simulink model "mc2_current_speed_fuzzy"  (R2023b)
settings: Solver=ode45  StartTime=0.0  StopTime=12  MaxStep=1e-5  RelTol=1e-3
libraries: spsDCVoltageSourceLib x2, spsUniversalBridgeLib x2, spsVoltageMeasurementLib x2, simulink x2, fuzblock x1, spspowerguiLib x1, sps_lib x1
settings Model: Creator=86189  LastModifiedBy=86189
settings SolverCC: ZeroCrossAlgorithm=Adaptive
settings DebuggingCC: IgnoredZcDiagnostic=none

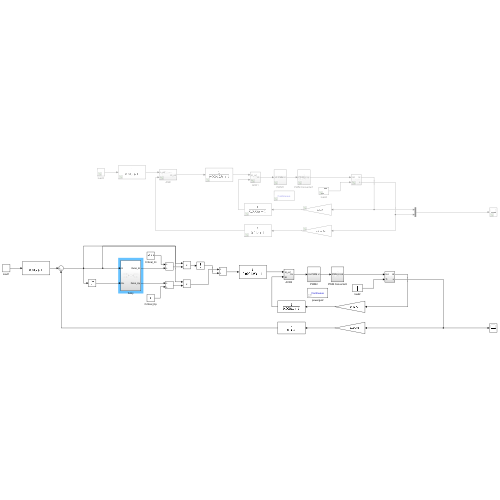
[thumbnail: Simulink's stored preview of the top-level diagram]
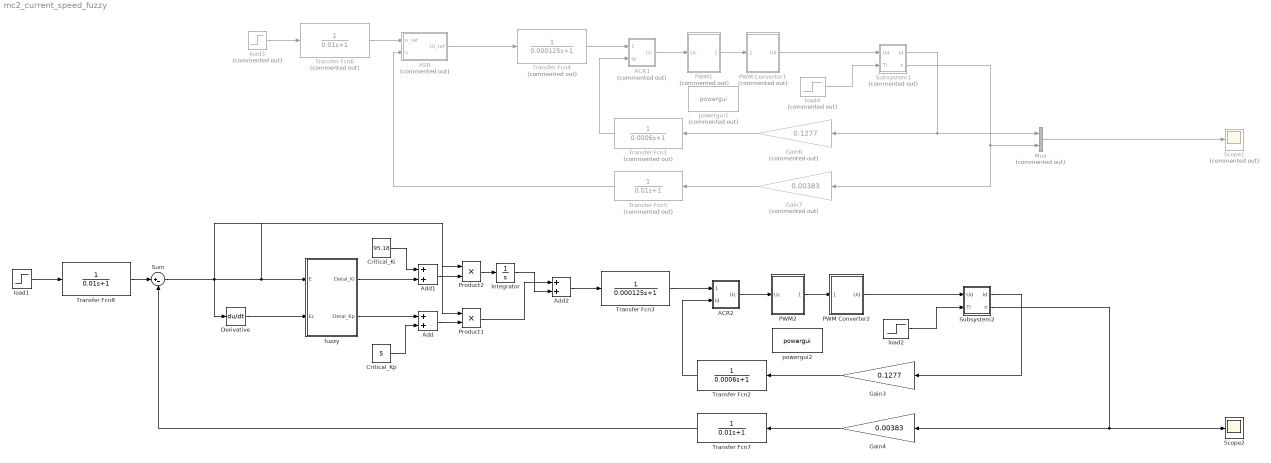
== system mc2_current_speed_fuzzy ==
  ACR1 : Subsystem  Commented=on
  ACR2 : Subsystem
  ASR : Subsystem  Commented=on
  Add : Sum
  Add1 : Sum
  Add2 : Sum
  Critical_Ki : Constant  Value=95.18
  Critical_Kp : Constant  Value=5
  Derivative : Derivative
  Gain3 : Gain  Gain=0.1277
  Gain4 : Gain  Gain=0.00383
  Gain6 : Gain  Commented=on  Gain=0.1277
  Gain7 : Gain  Commented=on  Gain=0.00383
  Integrator : Integrator
  Mux : Mux  Commented=on  Inputs=2
  PWM Converter1 : Subsystem  Commented=on
  PWM Converter2 : Subsystem
  PWM1 : Subsystem  Commented=on
  PWM2 : Subsystem
  Product1 : Product
  Product2 : Product
  Scope1 : Scope  Commented=on
  Scope2 : Scope
  Subsystem1 : Subsystem  Commented=on
  Subsystem2 : Subsystem
  Sum : Sum  Inputs=|+-
  Transfer Fcn1 : TransferFcn  Commented=on  Denominator=[0.0006 1]
  Transfer Fcn2 : TransferFcn  Denominator=[0.0006 1]
  Transfer Fcn3 : TransferFcn  Denominator=[0.000125 1]
  Transfer Fcn4 : TransferFcn  Commented=on  Denominator=[0.000125 1]
  Transfer Fcn5 : TransferFcn  Commented=on  Denominator=[0.01 1]
  Transfer Fcn6 : TransferFcn  Commented=on  Denominator=[0.01 1]
  Transfer Fcn7 : TransferFcn  Denominator=[0.01 1]
  Transfer Fcn8 : TransferFcn  Denominator=[0.01 1]
  fuzzy : Subsystem
  load1 : Step  Time=0  After=10  SampleTime=0
  load2 : Step  Time=0  After=0  SampleTime=0
  load3 : Step  Commented=on  Time=0  After=10  SampleTime=0
  load4 : Step  Commented=on  Time=0  After=0  SampleTime=0
  powergui1 : spspowerguiLib/powergui  Priority=1  Commented=on  SimulationMode=Continuous  SampleTime=50e-6  frequency=60  Iterations=50  frequencyindice=0  Pbase=100e6  ErrMax=1e-4  UnitsV=kV  UnitsW=MW  buscounter=0  FunctionMessages=off  echomessages=off  EnableUseOfTLC=off  CurrentSourceSwitches=off  DisableSnubberDevices=off  DisableRonSwitches=off  DisableVfSwitches=off  DisplayEquations=off  AutomaticDiscreteSolvers=off  SolverType=Tustin/Backward Euler (TBE)  Interpol=off  ExternalGateDelay=off  methode=off  Ts=100  x0status=blocks  SPID=on  SwTol=0  HookPort=off  NonlinearTolerance=1e-4  nMaxIteration=100  ContinueOnMaxIteration=off  RestoreLinks=warning  ResistiveCurrentMeasurement=off  Frange=[0:2:500]  Ylog=off  Xlog=on  ShowGrid=off  save=off  variable=ZData  structure=0  ZoomFFT=off  StartTime=0.0  cycles=1  DisplayStyle=1  fundamental=60  FreqAxis=off  MaxFrequency=1000  frequencyindicesteady=1  RmsSteady=1  display=off
  powergui2 : sps_lib/powergui  Priority=1  SimulationMode=Continuous  SampleTime=50e-6  frequency=60  Iterations=50  frequencyindice=0  Pbase=100e6  ErrMax=1e-4  UnitsV=kV  UnitsW=MW  buscounter=0  FunctionMessages=off  echomessages=off  EnableUseOfTLC=off  CurrentSourceSwitches=off  DisableSnubberDevices=off  DisableRonSwitches=off  DisableVfSwitches=off  DisplayEquations=off  AutomaticDiscreteSolvers=off  SolverType=Tustin/Backward Euler (TBE)  Interpol=off  ExternalGateDelay=off  methode=off  Ts=100  x0status=blocks  SPID=on  SwTol=0  HookPort=off  NonlinearTolerance=1e-4  nMaxIteration=100  ContinueOnMaxIteration=off  RestoreLinks=warning  ResistiveCurrentMeasurement=off  Frange=[0:2:500]  Ylog=off  Xlog=on  ShowGrid=off  save=off  variable=ZData  structure=0  ZoomFFT=off  StartTime=0.0  cycles=1  DisplayStyle=1  fundamental=60  FreqAxis=off  MaxFrequency=1000  frequencyindicesteady=1  RmsSteady=1  display=off
  wires:
  Transfer Fcn5/1 -> ASR/2(n)
  PWM1/1(PWM U) -> PWM Converter1/1(PWM U)
  ACR1/1(Uc) -> PWM1/1(Uc)
  load3/1 -> Transfer Fcn6/1
  Transfer Fcn6/1 -> ASR/1(n_ref)
  ASR/1(Ui_ref) -> Transfer Fcn4/1
  PWM Converter1/1(Ud) -> Subsystem1/1(Ud)
  Gain7/1 -> Transfer Fcn5/1
  Subsystem1/2(n) -> Mux/2, Gain7/1
  Transfer Fcn4/1 -> ACR1/1(Id_ref)
  Subsystem1/1(Id) -> Mux/1, Gain6/1
  load4/1 -> Subsystem1/2(Ti)
  Gain6/1 -> Transfer Fcn1/1
  Transfer Fcn1/1 -> ACR1/2(Id)
  Derivative/1 -> fuzzy/2(Ec)
  Critical_Kp/1 -> Add/2
  fuzzy/2(Detal_Kp) -> Add/1
  fuzzy/1(Detal_Ki) -> Add1/2
  Critical_Ki/1 -> Add1/1
  Integrator/1 -> Add2/2
  Transfer Fcn8/1 -> Sum/1
  Sum/1 -> Product1/1, Derivative/1, Product2/1, fuzzy/1(E)
  Add/1 -> Product1/2
  Add1/1 -> Product2/2
  Product2/1 -> Integrator/1
  Product1/1 -> Add2/1
  Add2/1 -> Transfer Fcn3/1
  load2/1 -> Subsystem2/2(Ti)
  Transfer Fcn2/1 -> ACR2/2(Id)
  Gain3/1 -> Transfer Fcn2/1
  load1/1 -> Transfer Fcn8/1
  Subsystem2/1(Id) -> Gain3/1
  Transfer Fcn3/1 -> ACR2/1(Id_ref)
  Subsystem2/2(n) -> Gain4/1, Scope2/1
  Gain4/1 -> Transfer Fcn7/1
  PWM2/1(PWM U) -> PWM Converter2/1(PWM U)
  ACR2/1(Uc) -> PWM2/1(Uc)
  PWM Converter2/1(Ud) -> Subsystem2/1(Ud)
  Transfer Fcn7/1 -> Sum/2
  Mux/1 -> Scope1/1

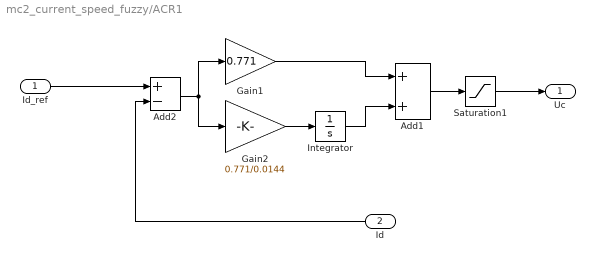
== system mc2_current_speed_fuzzy/ACR1 ==
  Id_ref : Inport
  Id : Inport  Port=2
  Add1 : Sum
  Add2 : Sum  Inputs=+-
  Gain1 : Gain  Gain=0.771
  Gain2 : Gain  Gain=0.771/0.0144
  Integrator : Integrator  LimitOutput=on  UpperSaturationLimit=5  LowerSaturationLimit=-5
  Saturation1 : Saturate  UpperLimit=5  LowerLimit=-5
  Uc : Outport
  wires:
  Gain2/1 -> Integrator/1
  Add1/1 -> Saturation1/1
  Integrator/1 -> Add1/2
  Add2/1 -> Gain2/1, Gain1/1
  Gain1/1 -> Add1/1
  Id/1 -> Add2/2
  Id_ref/1 -> Add2/1
  Saturation1/1 -> Uc/1

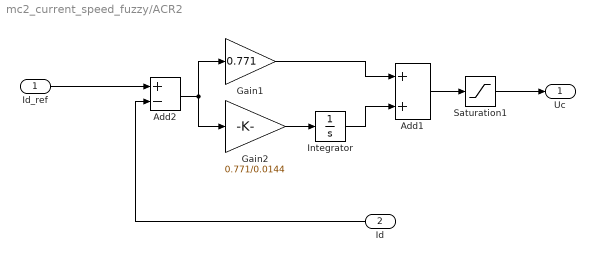
== system mc2_current_speed_fuzzy/ACR2 ==
  Id_ref : Inport
  Id : Inport  Port=2
  Add1 : Sum
  Add2 : Sum  Inputs=+-
  Gain1 : Gain  Gain=0.771
  Gain2 : Gain  Gain=0.771/0.0144
  Integrator : Integrator  LimitOutput=on  UpperSaturationLimit=5  LowerSaturationLimit=-5
  Saturation1 : Saturate  UpperLimit=5  LowerLimit=-5
  Uc : Outport
  wires:
  Gain2/1 -> Integrator/1
  Add1/1 -> Saturation1/1
  Integrator/1 -> Add1/2
  Add2/1 -> Gain2/1, Gain1/1
  Gain1/1 -> Add1/1
  Id/1 -> Add2/2
  Id_ref/1 -> Add2/1
  Saturation1/1 -> Uc/1

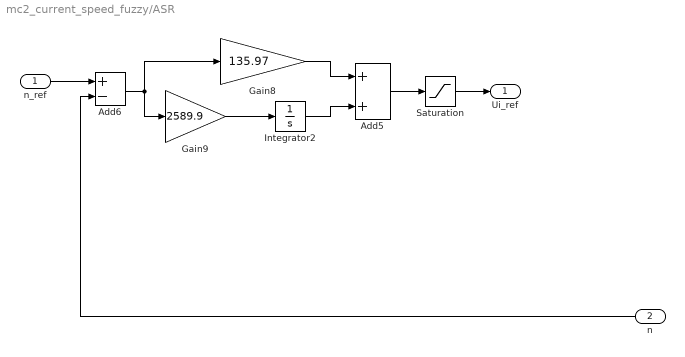
== system mc2_current_speed_fuzzy/ASR ==
  n_ref : Inport
  n : Inport  Port=2
  Add5 : Sum
  Add6 : Sum  Inputs=+-
  Gain8 : Gain  Gain=135.97
  Gain9 : Gain  Gain=2589.9
  Integrator2 : Integrator  LimitOutput=on  UpperSaturationLimit=5  LowerSaturationLimit=-5
  Saturation : Saturate  UpperLimit=5  LowerLimit=-5
  Ui_ref : Outport
  wires:
  Gain9/1 -> Integrator2/1
  n_ref/1 -> Add6/1
  Add6/1 -> Gain8/1, Gain9/1
  n/1 -> Add6/2
  Integrator2/1 -> Add5/2
  Gain8/1 -> Add5/1
  Add5/1 -> Saturation/1
  Saturation/1 -> Ui_ref/1

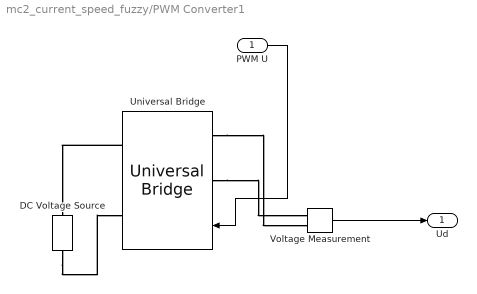
== system mc2_current_speed_fuzzy/PWM Converter1 ==
  PWM U : Inport
  DC Voltage Source : spsDCVoltageSourceLib/DC Voltage Source  Amplitude=538  Measurements=None
  Universal Bridge : spsUniversalBridgeLib/Universal Bridge  Arms=2  SnubberResistance=1e5  SnubberCapacitance=inf  Device=MOSFET / Diodes  Ron=1e-3  Lon=0  ForwardVoltages="[  0  0  ]"  ForwardVoltage=0  GTOparameters=[ 10e-6 , 20e-6 ]  IGBTparameters=[ 1e-6 , 2e-6 ]  Measurements=None  Measurements_2=None  converterType=Rectifier
  Voltage Measurement : spsVoltageMeasurementLib/Voltage Measurement  PhasorSimulation=off  OutputType=Complex  PSBequivalent=0
  Ud : Outport
  wires:
  PWM U/1 -> Universal Bridge/1
  Voltage Measurement/1 -> Ud/1
  connections:
  Universal Bridge/LConn2 -- Voltage Measurement/LConn2
  Universal Bridge/LConn1 -- Voltage Measurement/LConn1
  DC Voltage Source/RConn1 -- Universal Bridge/RConn1
  Universal Bridge/RConn2 -- DC Voltage Source/LConn1

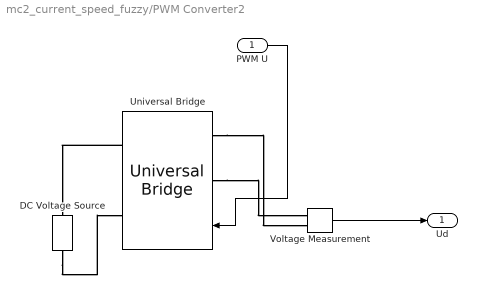
== system mc2_current_speed_fuzzy/PWM Converter2 ==
  PWM U : Inport
  DC Voltage Source : spsDCVoltageSourceLib/DC Voltage Source  Amplitude=538  Measurements=None
  Universal Bridge : spsUniversalBridgeLib/Universal Bridge  Arms=2  SnubberResistance=1e5  SnubberCapacitance=inf  Device=MOSFET / Diodes  Ron=1e-3  Lon=0  ForwardVoltages="[  0  0  ]"  ForwardVoltage=0  GTOparameters=[ 10e-6 , 20e-6 ]  IGBTparameters=[ 1e-6 , 2e-6 ]  Measurements=None  Measurements_2=None  converterType=Rectifier
  Voltage Measurement : spsVoltageMeasurementLib/Voltage Measurement  PhasorSimulation=off  OutputType=Complex  PSBequivalent=0
  Ud : Outport
  wires:
  PWM U/1 -> Universal Bridge/1
  Voltage Measurement/1 -> Ud/1
  connections:
  Universal Bridge/LConn2 -- Voltage Measurement/LConn2
  Universal Bridge/LConn1 -- Voltage Measurement/LConn1
  DC Voltage Source/RConn1 -- Universal Bridge/RConn1
  Universal Bridge/RConn2 -- DC Voltage Source/LConn1

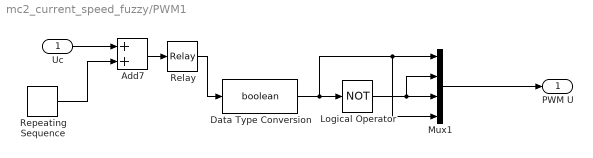
== system mc2_current_speed_fuzzy/PWM1 ==
  Uc : Inport
  Add7 : Sum
  Data Type Conversion : DataTypeConversion  OutDataTypeStr=boolean  SaturateOnIntegerOverflow=off  RndMeth=Floor
  Logical Operator : Logic  Operator=NOT  AllPortsSameDT=off  OutDataTypeStr=boolean
  Mux1 : Mux
      settings: DisplayOption=signals
  Relay : Relay  OnSwitchValue=0  OffSwitchValue=0
  Repeating Sequence : simulink/Sources/Repeating Sequence  rep_seq_t=[0 0.125e-3]  rep_seq_y=[-5 5]
  PWM U : Outport
  wires:
  Repeating Sequence/1 -> Add7/2
  Data Type Conversion/1 -> Mux1/4, Mux1/1, Logical Operator/1
  Logical Operator/1 -> Mux1/2, Mux1/3
  Add7/1 -> Relay/1
  Mux1/1 -> PWM U/1
  Relay/1 -> Data Type Conversion/1
  Uc/1 -> Add7/1

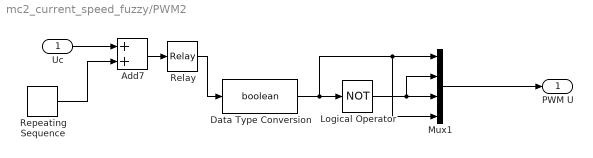
== system mc2_current_speed_fuzzy/PWM2 ==
  Uc : Inport
  Add7 : Sum
  Data Type Conversion : DataTypeConversion  OutDataTypeStr=boolean  SaturateOnIntegerOverflow=off  RndMeth=Floor
  Logical Operator : Logic  Operator=NOT  AllPortsSameDT=off  OutDataTypeStr=boolean
  Mux1 : Mux
      settings: DisplayOption=signals
  Relay : Relay  OnSwitchValue=0  OffSwitchValue=0
  Repeating Sequence : simulink/Sources/Repeating Sequence  rep_seq_t=[0 0.125e-3]  rep_seq_y=[-5 5]
  PWM U : Outport
  wires:
  Repeating Sequence/1 -> Add7/2
  Data Type Conversion/1 -> Mux1/4, Mux1/1, Logical Operator/1
  Logical Operator/1 -> Mux1/2, Mux1/3
  Add7/1 -> Relay/1
  Mux1/1 -> PWM U/1
  Relay/1 -> Data Type Conversion/1
  Uc/1 -> Add7/1

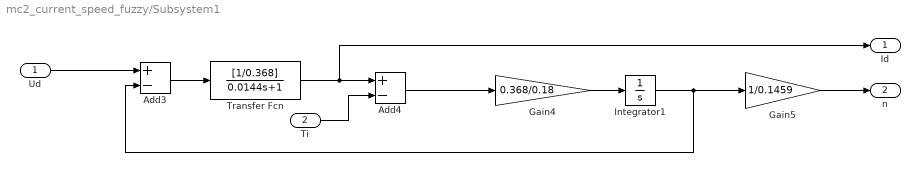
== system mc2_current_speed_fuzzy/Subsystem1 ==
  Ud : Inport
  Ti : Inport  Port=2
  Add3 : Sum  Inputs=+-
  Add4 : Sum  Inputs=+-
  Gain4 : Gain  Gain=0.368/0.18
  Gain5 : Gain  Gain=1/0.1459
  Integrator1 : Integrator
  Transfer Fcn : TransferFcn  Numerator=[1/0.368]  Denominator=[0.0144 1]
  Id : Outport
  n : Outport  Port=2
  wires:
  Add3/1 -> Transfer Fcn/1
  Transfer Fcn/1 -> Id/1, Add4/1
  Ud/1 -> Add3/1
  Add4/1 -> Gain4/1
  Integrator1/1 -> Add3/2, Gain5/1
  Gain4/1 -> Integrator1/1
  Gain5/1 -> n/1
  Ti/1 -> Add4/2

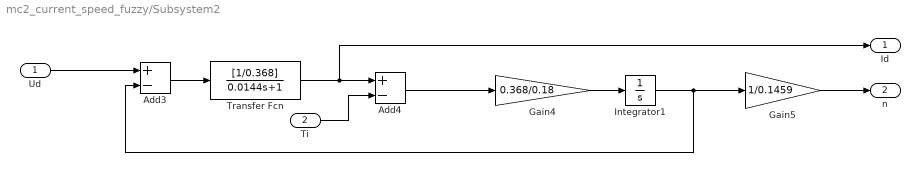
== system mc2_current_speed_fuzzy/Subsystem2 ==
  Ud : Inport
  Ti : Inport  Port=2
  Add3 : Sum  Inputs=+-
  Add4 : Sum  Inputs=+-
  Gain4 : Gain  Gain=0.368/0.18
  Gain5 : Gain  Gain=1/0.1459
  Integrator1 : Integrator
  Transfer Fcn : TransferFcn  Numerator=[1/0.368]  Denominator=[0.0144 1]
  Id : Outport
  n : Outport  Port=2
  wires:
  Add3/1 -> Transfer Fcn/1
  Transfer Fcn/1 -> Id/1, Add4/1
  Ud/1 -> Add3/1
  Add4/1 -> Gain4/1
  Integrator1/1 -> Add3/2, Gain5/1
  Gain4/1 -> Integrator1/1
  Gain5/1 -> n/1
  Ti/1 -> Add4/2

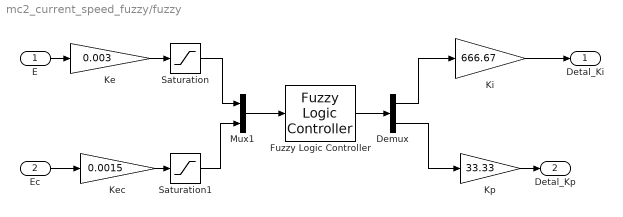
== system mc2_current_speed_fuzzy/fuzzy ==
  E : Inport
  Ec : Inport  Port=2
  Demux : Demux  Outputs=2
  Fuzzy Logic Controller : fuzblock/Fuzzy Logic  Controller  FIS='FuzzyPI.fis'  OutputSampleNumber=101  DataType=double  FuzzifiedInputs=off  RuleFiringStrengths=off  RuleOutputs=off  AggregatedOutputs=off  SimulateUsing=Interpreted execution  OutOfRangeInputValueMessage=warning  NoRuleFiredMessage=warning  EmptyOutputFuzzySetMessage=warning
  Ke : Gain  Gain=0.003
  Kec : Gain  Gain=0.0015
  Ki : Gain  Gain=666.67
  Kp : Gain  Gain=33.33
  Mux1 : Mux  Inputs=2
  Saturation : Saturate
  Saturation1 : Saturate
  Detal_Ki : Outport
  Detal_Kp : Outport  Port=2
  wires:
  Kec/1 -> Saturation1/1
  Demux/2 -> Kp/1
  Ec/1 -> Kec/1
  Demux/1 -> Ki/1
  Mux1/1 -> Fuzzy Logic Controller/1
  Ki/1 -> Detal_Ki/1
  Fuzzy Logic Controller/1 -> Demux/1
  Saturation/1 -> Mux1/1
  Kp/1 -> Detal_Kp/1
  E/1 -> Ke/1
  Ke/1 -> Saturation/1
  Saturation1/1 -> Mux1/2
